simulink model "soc_image_rotation_fpga"  (R2025a)
settings: Solver=FixedStepAuto  StartTime=0.0  StopTime=10.0  RelTol=1e-3
undefined symbols (not defined in the file or in its folder): bytesPerPixel, imageHeight, imageWidth
libraries: hwlogicconnlib x4, hdlsllib x1
settings Model: Creator=The MathWorks, Inc.  LastModifiedBy=The MathWorks, Inc.
settings SolverCC: AlgebraicLoopSolver=TrustRegion
settings DataIOCC: SaveOutput=off  SaveTime=off  ReturnWorkspaceOutputs=off
settings OptimizationCC: DefaultParameterBehavior=Inlined  ReuseModelBlockBuffer=off
settings DebuggingCC: UnconnectedInputMsg=warning  UnconnectedOutputMsg=warning  UnconnectedLineMsg=warning  ArithmeticOperatorsInVariantConditions=warning
settings HardwareCC: ProdBitPerPointer=32.0  ProdBitPerSizeT=32.0  ProdBitPerPtrDiffT=32.0  ProdLargestAtomicFloat=None  ProdIntDivRoundTo=Undefined  ProdEndianess=Unspecified  ProdWordSize=32.0  ProdHWDeviceType=ASIC/FPGA->ASIC/FPGA  TargetBitPerLong=64.0  TargetBitPerPointer=64.0  TargetBitPerSizeT=64.0  TargetBitPerPtrDiffT=64.0  TargetLongLongMode=on  TargetIntDivRoundTo=Zero  TargetEndianess=LittleEndian  TargetWordSize=64.0  TargetHWDeviceType=Custom Processor->MATLAB Host Computer  ProdEqTarget=off
settings ModelReferenceCC: EnableRefExpFcnMdlSchedulingChecks=on  ModelReferenceNumInstancesAllowed=Single
settings SFSimCC: SimUseLocalCustomCode=off
settings RTWCC: RTWUseLocalCustomCode=off  GPUComputeCapability=3.5  DLArmComputeVersion=19.05
settings GRTTargetCC: CombineOutputUpdateFcns=off  MatFileLogging=off  SubcomponentCodeInterfacePackaging=Nonreusable function

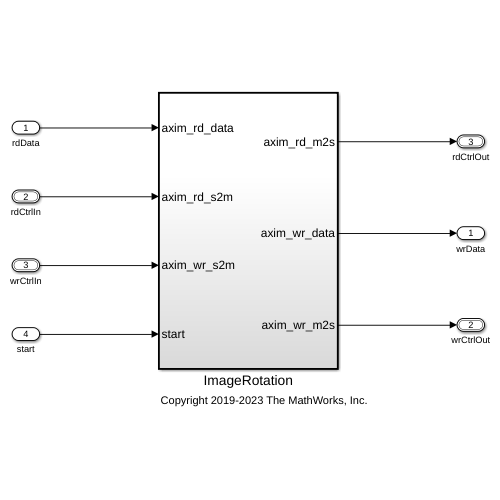
[thumbnail: Simulink's stored preview of the top-level diagram]
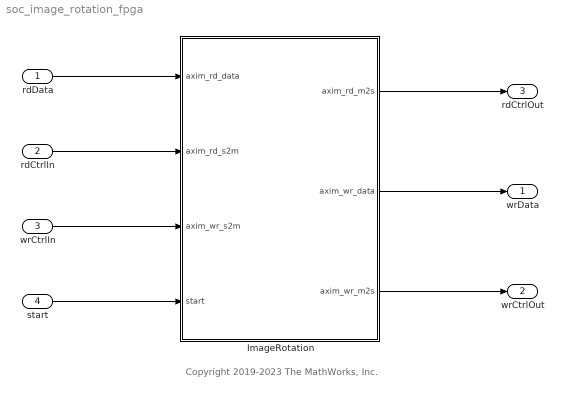
== system soc_image_rotation_fpga ==
  note: Copyright 2019-2023 The MathWorks, Inc.
  rdData : Inport  OutDataTypeStr=dt  SampleTime=[1.9999999999999999e-06,0]
  rdCtrlIn : Inport  Port=2  OutDataTypeStr=Bus: ReadControlS2MBusObj  SampleTime=[1.9999999999999999e-06,0]  BusOutputAsStruct=on
  wrCtrlIn : Inport  Port=3  OutDataTypeStr=Bus: WriteControlS2MBusObj  SampleTime=[1.9999999999999999e-06,0]  BusOutputAsStruct=on
  start : Inport  Port=4  OutDataTypeStr=boolean  SampleTime=[1.9999999999999999e-06,0]
  ImageRotation : Subsystem  TreatAsAtomicUnit=on
  wrData : Outport  OutDataTypeStr=dt  PortDimensions=1  SampleTime=[1.9999999999999999e-06,0]  VectorParamsAs1DForOutWhenUnconnected=off
  wrCtrlOut : Outport  Port=2  OutDataTypeStr=Bus: WriteControlM2SBusObj  PortDimensions=1  SampleTime=[1.9999999999999999e-06,0]  VectorParamsAs1DForOutWhenUnconnected=off  BusOutputAsStruct=on
  rdCtrlOut : Outport  Port=3  OutDataTypeStr=Bus: ReadControlM2SBusObj  PortDimensions=1  SampleTime=[1.9999999999999999e-06,0]  VectorParamsAs1DForOutWhenUnconnected=off  BusOutputAsStruct=on
  wires:
  ImageRotation/3(axim_wr_m2s) -> wrCtrlOut/1
  start/1 -> ImageRotation/4(start)
  ImageRotation/1(axim_rd_m2s) -> rdCtrlOut/1
  wrCtrlIn/1 -> ImageRotation/3(axim_wr_s2m)
  rdCtrlIn/1 -> ImageRotation/2(axim_rd_s2m)
  rdData/1 -> ImageRotation/1(axim_rd_data)
  ImageRotation/2(axim_wr_data) -> wrData/1

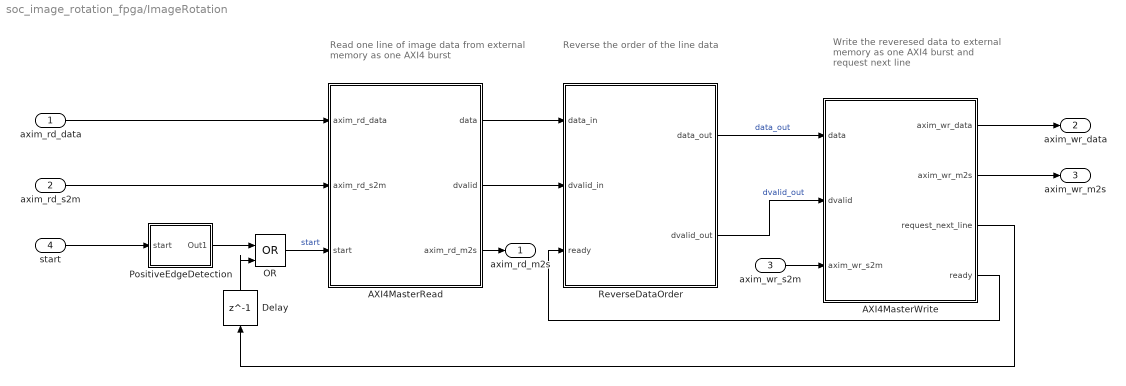
== system soc_image_rotation_fpga/ImageRotation ==
  note: Read one line of image data from external memory as one AXI4 burst
  note: Write the reveresed data to external memory as one AXI4 burst and request next line
  note: Reverse the order of the line data
  axim_rd_data : Inport
  axim_rd_s2m : Inport  Port=2
  axim_wr_s2m : Inport  Port=3
  start : Inport  Port=4
  AXI4MasterRead : Subsystem
  AXI4MasterWrite : Subsystem
  Delay : Delay  DelayLength=1
  OR : Logic  Operator=OR  IconShape=distinctive  AllPortsSameDT=off  OutDataTypeStr=boolean
  PositiveEdgeDetection : Subsystem
  ReverseDataOrder : Subsystem
  axim_rd_m2s : Outport  VectorParamsAs1DForOutWhenUnconnected=off
  axim_wr_data : Outport  Port=2  VectorParamsAs1DForOutWhenUnconnected=off
  axim_wr_m2s : Outport  Port=3  VectorParamsAs1DForOutWhenUnconnected=off
  wires:
  axim_rd_s2m/1 -> AXI4MasterRead/2(axim_rd_s2m)
  ReverseDataOrder/2(dvalid_out) -> AXI4MasterWrite/2(dvalid)  "dvalid_out"
  ReverseDataOrder/1(data_out) -> AXI4MasterWrite/1(data)  "data_out"
  axim_rd_data/1 -> AXI4MasterRead/1(axim_rd_data)
  OR/1 -> AXI4MasterRead/3(start)  "start"
  AXI4MasterRead/3(axim_rd_m2s) -> axim_rd_m2s/1
  AXI4MasterRead/1(data) -> ReverseDataOrder/1(data_in)
  AXI4MasterRead/2(dvalid) -> ReverseDataOrder/2(dvalid_in)
  AXI4MasterWrite/4(ready) -> ReverseDataOrder/3(ready)
  AXI4MasterWrite/2(axim_wr_m2s) -> axim_wr_m2s/1
  axim_wr_s2m/1 -> AXI4MasterWrite/3(axim_wr_s2m)
  PositiveEdgeDetection/1(Out1) -> OR/1
  Delay/1 -> OR/2
  AXI4MasterWrite/3(request_next_line) -> Delay/1
  AXI4MasterWrite/1(axim_wr_data) -> axim_wr_data/1
  start/1 -> PositiveEdgeDetection/1(start)

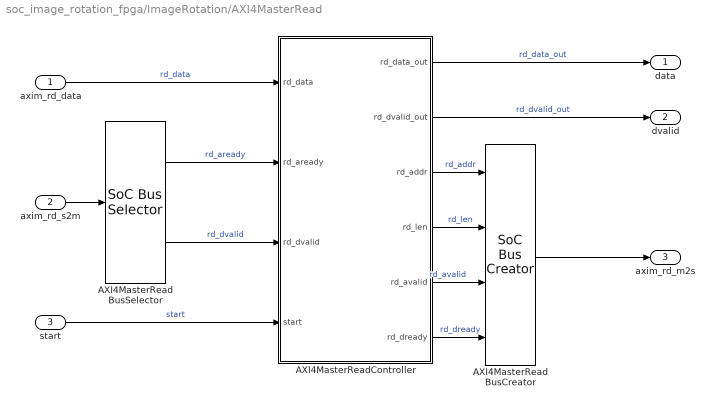
== system soc_image_rotation_fpga/ImageRotation/AXI4MasterRead ==
  axim_rd_data : Inport
  axim_rd_s2m : Inport  Port=2
  start : Inport  Port=3
  AXI4MasterRead BusCreator : hwlogicconnlib/SoC Bus Creator  Protocol=Random access read  ctrltype=Ready
  AXI4MasterRead BusSelector : hwlogicconnlib/SoC Bus Selector  Protocol=Random access read  ctrltype=Valid
  AXI4MasterReadController : MATLAB Function  TreatAsAtomicUnit=on
  data : Outport  VectorParamsAs1DForOutWhenUnconnected=off
  dvalid : Outport  Port=2  VectorParamsAs1DForOutWhenUnconnected=off
  axim_rd_m2s : Outport  Port=3  VectorParamsAs1DForOutWhenUnconnected=off
  wires:
  start/1 -> AXI4MasterReadController/4(start)  "start"
  AXI4MasterReadController/4(rd_len) -> AXI4MasterRead BusCreator/2  "rd_len"
  AXI4MasterReadController/3(rd_addr) -> AXI4MasterRead BusCreator/1  "rd_addr"
  axim_rd_s2m/1 -> AXI4MasterRead BusSelector/1
  AXI4MasterRead BusSelector/2 -> AXI4MasterReadController/3(rd_dvalid)  "rd_dvalid"
  AXI4MasterRead BusSelector/1 -> AXI4MasterReadController/2(rd_aready)  "rd_aready"
  AXI4MasterReadController/2(rd_dvalid_out) -> dvalid/1  "rd_dvalid_out"
  AXI4MasterReadController/1(rd_data_out) -> data/1  "rd_data_out"
  axim_rd_data/1 -> AXI4MasterReadController/1(rd_data)  "rd_data"
  AXI4MasterReadController/5(rd_avalid) -> AXI4MasterRead BusCreator/3  "rd_avalid"
  AXI4MasterReadController/6(rd_dready) -> AXI4MasterRead BusCreator/4  "rd_dready"
  AXI4MasterRead BusCreator/1 -> axim_rd_m2s/1

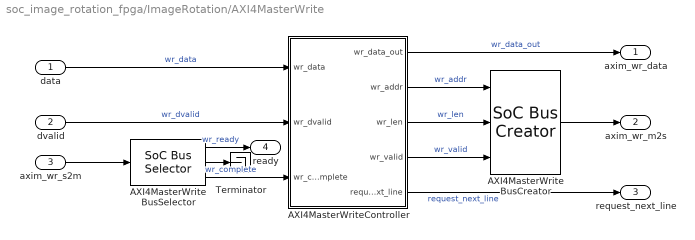
== system soc_image_rotation_fpga/ImageRotation/AXI4MasterWrite ==
  data : Inport
  dvalid : Inport  Port=2
  axim_wr_s2m : Inport  Port=3
  AXI4MasterWrite BusCreator : hwlogicconnlib/SoC Bus Creator  Protocol=Random access write  ctrltype=Valid
  AXI4MasterWrite BusSelector : hwlogicconnlib/SoC Bus Selector  Protocol=Random access write  ctrltype=Ready
  AXI4MasterWriteController : MATLAB Function  TreatAsAtomicUnit=on
  Terminator : Terminator
  axim_wr_data : Outport  VectorParamsAs1DForOutWhenUnconnected=off
  axim_wr_m2s : Outport  Port=2  VectorParamsAs1DForOutWhenUnconnected=off
  request_next_line : Outport  Port=3  VectorParamsAs1DForOutWhenUnconnected=off
  ready : Outport  Port=4  VectorParamsAs1DForOutWhenUnconnected=off
  wires:
  AXI4MasterWriteController/1(wr_data_out) -> axim_wr_data/1  "wr_data_out"
  AXI4MasterWriteController/3(wr_len) -> AXI4MasterWrite BusCreator/2  "wr_len"
  dvalid/1 -> AXI4MasterWriteController/2(wr_dvalid)  "wr_dvalid"
  AXI4MasterWriteController/4(wr_valid) -> AXI4MasterWrite BusCreator/3  "wr_valid"
  AXI4MasterWrite BusSelector/2 -> Terminator/1
  AXI4MasterWriteController/2(wr_addr) -> AXI4MasterWrite BusCreator/1  "wr_addr"
  axim_wr_s2m/1 -> AXI4MasterWrite BusSelector/1
  AXI4MasterWrite BusCreator/1 -> axim_wr_m2s/1
  AXI4MasterWriteController/5(request_next_line) -> request_next_line/1  "request_next_line"
  AXI4MasterWrite BusSelector/1 -> ready/1  "wr_ready"
  AXI4MasterWrite BusSelector/3 -> AXI4MasterWriteController/3(wr_complete)  "wr_complete"
  data/1 -> AXI4MasterWriteController/1(wr_data)  "wr_data"

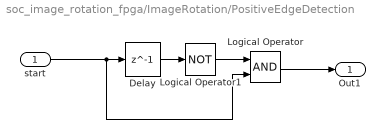
== system soc_image_rotation_fpga/ImageRotation/PositiveEdgeDetection ==
  start : Inport
  Delay : Delay  DelayLength=1
  Logical Operator : Logic  AllPortsSameDT=off  OutDataTypeStr=boolean
  Logical Operator1 : Logic  Operator=NOT  AllPortsSameDT=off  OutDataTypeStr=boolean
  Out1 : Outport  VectorParamsAs1DForOutWhenUnconnected=off
  wires:
  start/1 -> Logical Operator/2, Delay/1
  Delay/1 -> Logical Operator1/1
  Logical Operator1/1 -> Logical Operator/1
  Logical Operator/1 -> Out1/1

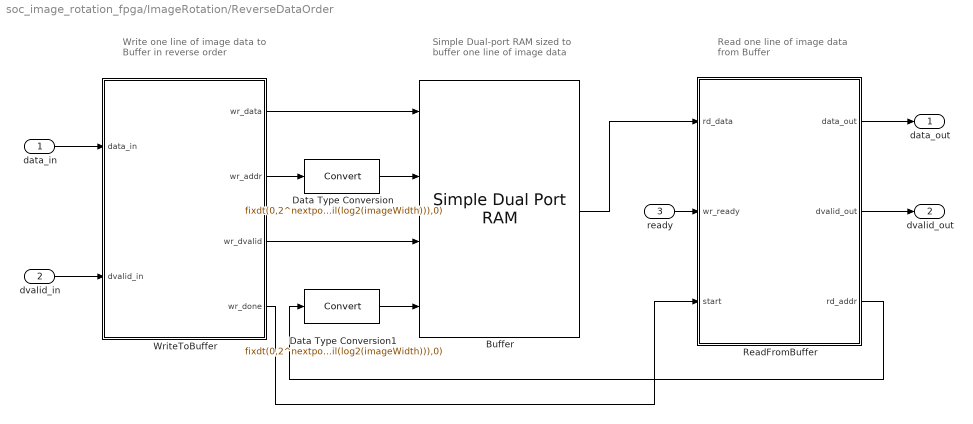
== system soc_image_rotation_fpga/ImageRotation/ReverseDataOrder ==
  note: Write one line of image data to Buffer in reverse order
  note: Read one line of image data from Buffer
  note: Simple Dual-port RAM sized to buffer one line of image data
  data_in : Inport
  dvalid_in : Inport  Port=2
  ready : Inport  Port=3
  Buffer : hdlsllib/HDL RAMs/Simple Dual Port RAM  ram_size=2^nextpow2(ceil(log2(imageWidth)))
  Data Type Conversion : DataTypeConversion  OutDataTypeStr=fixdt(0,2^nextpow2(ceil(log2(imageWidth))),0)  SaturateOnIntegerOverflow=off  RndMeth=Floor
  Data Type Conversion1 : DataTypeConversion  OutDataTypeStr=fixdt(0,2^nextpow2(ceil(log2(imageWidth))),0)  SaturateOnIntegerOverflow=off  RndMeth=Floor
  ReadFromBuffer : MATLAB Function  TreatAsAtomicUnit=on
  WriteToBuffer : MATLAB Function  TreatAsAtomicUnit=on
  data_out : Outport  VectorParamsAs1DForOutWhenUnconnected=off
  dvalid_out : Outport  Port=2  VectorParamsAs1DForOutWhenUnconnected=off
  wires:
  ReadFromBuffer/2(dvalid_out) -> dvalid_out/1
  dvalid_in/1 -> WriteToBuffer/2(dvalid_in)
  ReadFromBuffer/3(rd_addr) -> Data Type Conversion1/1
  ReadFromBuffer/1(data_out) -> data_out/1
  WriteToBuffer/3(wr_dvalid) -> Buffer/3
  WriteToBuffer/1(wr_data) -> Buffer/1
  WriteToBuffer/2(wr_addr) -> Data Type Conversion/1
  data_in/1 -> WriteToBuffer/1(data_in)
  Buffer/1 -> ReadFromBuffer/1(rd_data)
  ready/1 -> ReadFromBuffer/2(wr_ready)
  WriteToBuffer/4(wr_done) -> ReadFromBuffer/3(start)
  Data Type Conversion/1 -> Buffer/2
  Data Type Conversion1/1 -> Buffer/4

== matlab function soc_image_rotation_fpga/ImageRotation/AXI4MasterWrite/AXI4MasterWriteController ==
  data: wr_data_out output; wr_addr output; wr_len output; wr_valid output; request_next_line output; wr_data input; wr_dvalid input; wr_complete input; imageWidth parameter; imageHeight parameter; bytesPerPixel parameter
function [wr_data_out, wr_addr,wr_len, wr_valid, request_next_line] = fcn(wr_data, wr_dvalid, wr_complete, imageWidth, imageHeight, bytesPerPixel)
% Finite State Machine (FSM) for AXI4 Master Write Controller

% Copyright 2018 The MathWorks, Inc.

% Create persistent variables (registers)
persistent burst_count;
if(isempty(burst_count))
    burst_count = uint32(0);
end
persistent line_count;
if(isempty(line_count))
    line_count = uint32(0);
end

% State Memory Encoding
IDLE              = uint32(0);
DATA_COUNT        = uint32(1);

persistent wstate;
if(isempty(wstate))
    wstate = IDLE;
end

% Write lines of image data in the reversed order. 
% One line takes imageWidth*bytesPerPixel bytes. 
% wr_addr decreases by imageWidth*bytesPerPixel for each write burst
wr_addr = uint32(imageWidth*bytesPerPixel*(imageHeight-1)- line_count*imageWidth*bytesPerPixel);

% send one line (fixed length) for each write burst
wr_len = uint32(imageWidth);

wr_valid = wr_dvalid ;
wr_data_out = wr_data;

% FSM for AXI4Master Write
switch (wstate)
    case IDLE
        if ( wr_dvalid )
            wstate = DATA_COUNT;
            burst_count = uint32(burst_count + 1); % count incoming samples
        else
            wstate = IDLE;
        end
    case DATA_COUNT
        % State vars
        if ( burst_count == uint32(imageWidth) )
            wstate = IDLE;
            burst_count = uint32(0);
            % increase line_count until it reaches imageHeight after each burst
            if line_count == uint32(imageHeight-1)
                line_count = uint32(0);
            else
                line_count = uint32(line_count +1);
            end
        else
            burst_count = burst_count + uint32(wr_dvalid);
        end 
    otherwise
        wstate = IDLE;
end

% request next line if wr_complete is high
% And no request after last line write is finished.
request_next_line = wr_complete && (line_count ~= 0); 

end

== matlab function soc_image_rotation_fpga/ImageRotation/ReverseDataOrder/ReadFromBuffer ==
  data: rd_data input; wr_ready input; data_out output; dvalid_out output boolean; start input boolean; rd_addr output; imageWidth parameter
function [data_out,dvalid_out, rd_addr] = fcn(rd_data,wr_ready, start, imageWidth)
% read data from buffer in order

% Copyright 2018 The MathWorks, Inc.

% Create persistent variables (registers)
persistent burst_count;
if(isempty(burst_count))
    burst_count = uint16(0);
end

% State Memory Encoding
IDLE        = uint32(0);
WAIT_WREADY = uint32(1);
DATA_COUNT  = uint32(2);

persistent rstate;
if(isempty(rstate))
    rstate = IDLE;
end

persistent dvalid_d; % davlid_d is dvalid delayed by one clock cycle
if(isempty(dvalid_d))
    dvalid_d = false;
end

data_out = rd_data;
dvalid_out = dvalid_d;
rd_addr = burst_count;

% FSM for buffer reading
switch (rstate)
    case IDLE
        dvalid = false;
        burst_count = uint16(0);
        if start % reading starts when 'start' signal is received
            rstate = WAIT_WREADY;
        end
    case WAIT_WREADY
        dvalid = false;
        if wr_ready
            rstate = DATA_COUNT;
        end
    case DATA_COUNT
        if wr_ready % counting when wr_ready is high
            dvalid = true;
            if ( burst_count == uint16(imageWidth-1)) % go to IDLE when counting is done
                rstate = IDLE;
            else
                burst_count = burst_count + 1;
            end
        else
            dvalid = false;
            rstate = DATA_COUNT;
        end
    otherwise
        dvalid = false;
        rstate = IDLE;
end

dvalid_d = dvalid; % delay dvalid for one cycle to sync with rd_data
end

== matlab function soc_image_rotation_fpga/ImageRotation/AXI4MasterRead/AXI4MasterReadController ==
  data: rd_data input; rd_aready input; rd_dvalid input; rd_data_out output; rd_dvalid_out output; start input; rd_addr output; rd_len output; rd_avalid output; imageWidth parameter; imageHeight parameter; bytesPerPixel parameter; rd_dready output
function [rd_data_out, rd_dvalid_out, rd_addr, rd_len, rd_avalid, rd_dready] = fcn(rd_data, rd_aready, rd_dvalid, start, imageWidth, imageHeight, bytesPerPixel)
% Finite State Machine (FSM) for AXI4 Master Read Controller

% Copyright 2018 The MathWorks, Inc.

% Create persistent variables (registers)
persistent burst_count;
if(isempty(burst_count))
    burst_count = uint32(0);
end

persistent line_count;
if(isempty(line_count))
    line_count = uint32(0);
end

% State Encoding
IDLE             = uint32(0);
READ_BURST_START = uint32(1);
DATA_COUNT       = uint32(2);

persistent rstate;
if isempty(rstate)
    rstate = IDLE;
end

% one line takes imageWidth*bytesPerPixel bytes 
% rd_addr increases by imageWidth*bytesPerPixel for each read burst
rd_addr = uint32(imageWidth*bytesPerPixel*line_count);

% request one line (fixed length) for each read burst
rd_len = uint32(imageWidth);

% rd_dready is always high as no backpress signal from downstream
rd_dready = true;

rd_data_out = rd_data;
rd_dvalid_out = rd_dvalid;

% FSM for AXI4Master Read
switch (rstate)      
    case IDLE
        rd_avalid = false;
        burst_count = uint32(0); % reset burst count        
        if start
            rstate = READ_BURST_START;
        end
    case READ_BURST_START
        if rd_aready % when rd_aready is high, send read request by asserting rd_avalid
            rd_avalid = true; 
            rstate = DATA_COUNT;
        else % wait when rd_aready is low
            rd_avalid = false;
            rstate = READ_BURST_START;
        end
    case DATA_COUNT
        rd_avalid = false; % de-aserrt rd_avalid when reading data
        burst_count = burst_count + uint32(rd_dvalid); % count incoming samples
        if burst_count == rd_len
            rstate = IDLE; % go to IDLE state when burst_count reaches imageWidth
            % increase line_count until it reaches imageHeight after each burst
            if line_count == uint32(imageHeight -1) 
                line_count = uint32(0);
            else 
                line_count = uint32(line_count + 1);
            end
        end
    otherwise
        rd_avalid = false;
        rstate = IDLE;
end

== matlab function soc_image_rotation_fpga/ImageRotation/ReverseDataOrder/WriteToBuffer ==
  data: wr_data output; wr_addr output; wr_dvalid output; data_in input; dvalid_in input; wr_done output; imageWidth parameter
function [wr_data,wr_addr, wr_dvalid, wr_done] = fcn(data_in, dvalid_in, imageWidth)
% Write data to buffer in reverse order

% Copyright 2018 The MathWorks, Inc.

% Create persistent variables (registers)
persistent burst_count;
if(isempty(burst_count))
    burst_count = uint16(imageWidth-1); % countdown from (imageWidth-1) to 0
end

wr_data = data_in;
wr_dvalid = dvalid_in;
wr_addr = burst_count;
wr_done = (burst_count == uint16(0)) && dvalid_in; % wr_done asserts after burst_count reaches 0

% State vars
if ( dvalid_in )
    if ( burst_count == uint16(0) )
        burst_count = uint16(imageWidth-1); % reset to imageWidth-1 for next line
    else
        burst_count = uint16(burst_count - 1);
    end
end

end
